simulink model "simulink_4_balloons"  (R2020b)
settings: Solver=VariableStepAuto  StartTime=0.0  StopTime=300  RelTol=1e-3
InitFcn:
  | seed1 = randi(100000);
  | seed2 = randi(200000);
values from neighbouring files (symbols this model uses):
  Cd = 0.418    [sim_4balloon_test.m]
  mb1 = 3/1000    (= 0.003)    [sim_4balloon_test.m]
  mb2 = 3/1000    (= 0.003)    [sim_4balloon_test.m]
  mb3 = 3/1000    (= 0.003)    [sim_4balloon_test.m]
  mb4 = 3/1000    (= 0.003)    [sim_4balloon_test.m]
  nH = x(2)    [sim_4balloon_test.m]
  normalScaling = x(5)    [sim_4balloon_test.m]
  nS = x(3)    [sim_4balloon_test.m]
  nV = x(1)    [sim_4balloon_test.m]
  rb = 80/1000    (= 0.08)    [sim_4balloon_test.m]
  rb1 = 80/1000    (= 0.08)    [sim_4balloon_test.m]
  rb2 = 80/1000    (= 0.08)    [sim_4balloon_test.m]
  rb3 = 80/1000    (= 0.08)    [sim_4balloon_test.m]
  rb4 = 80/1000    (= 0.08)    [sim_4balloon_test.m]
  rn = 125/2000    (= 0.0625)    [sim_4balloon_test.m]
  seedX1 = randi(100000)    [sim_4balloon_test.m]
  seedX2 = randi(100000)    [sim_4balloon_test.m]
  seedX3 = randi(100000)    [sim_4balloon_test.m]
  seedX4 = randi(100000)    [sim_4balloon_test.m]
  seedY1 = randi(100000)    [sim_4balloon_test.m]
  seedY2 = randi(100000)    [sim_4balloon_test.m]
  seedY3 = randi(100000)    [sim_4balloon_test.m]
  seedY4 = randi(100000)    [sim_4balloon_test.m]
  seedZ1 = randi(100000)    [sim_4balloon_test.m]
  seedZ2 = randi(100000)    [sim_4balloon_test.m]
  seedZ3 = randi(100000)    [sim_4balloon_test.m]
  seedZ4 = randi(100000)    [sim_4balloon_test.m]
  theta = x(7)    [sim_4balloon_test.m]
  V0 = x(4)    [sim_4balloon_test.m]
undefined symbols (not defined in the file or in its folder): coefficient_dragq, coefficient_sideforceq
libraries: nesl_utility x41, sm_lib x25, eeGeneralControl x12
(part 2 of 2)

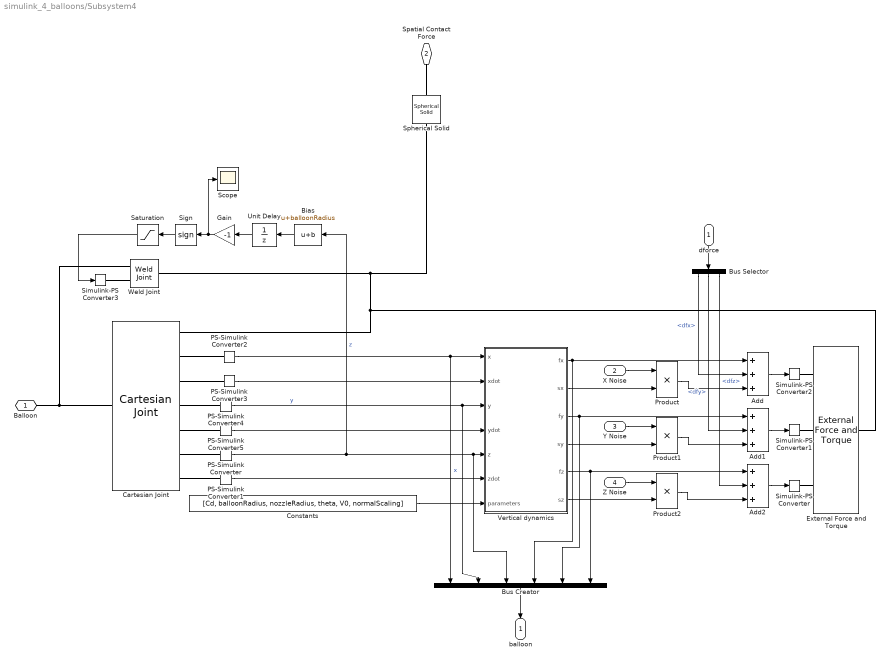
== system simulink_4_balloons/Subsystem4 ==
  dforce : Inport
  X Noise : Inport  Port=2
  Y Noise : Inport  Port=3
  Z Noise : Inport  Port=4
  Add : Sum  Inputs=+++
  Add1 : Sum  Inputs=+++
  Add2 : Sum  Inputs=+++
  Bias : Bias  Bias=balloonRadius
  Bus Creator : BusCreator  Inputs=6
  Bus Selector : BusSelector  OutputSignals=dfx,dfy,dfz
  Cartesian Joint : sm_lib/Joints/Cartesian Joint  JointMode=Normal  SenseConstraintForce=off  SenseConstraintForceX=off  SenseConstraintForceY=off  SenseConstraintForceZ=off  SenseConstraintTorque=off  SenseConstraintTorqueX=off  SenseConstraintTorqueY=off  SenseConstraintTorqueZ=off  SenseTotalForce=off  SenseTotalForceX=off  SenseTotalForceY=off  SenseTotalForceZ=off  SenseTotalTorque=off  SenseTotalTorqueX=off  SenseTotalTorqueY=off  SenseTotalTorqueZ=off  CompositeWrenchDir=FollowerOnBase  CompositeWrenchFrame=BaseFrame  PxEquilibriumPosition=0  PxEquilibriumPositionUnits=m  PxSpringStiffness=0  PxSpringStiffnessUnits=N/m  PxDampingCoefficient=hd  PxDampingCoefficientUnits=N/(m/s)  PxTorqueActuationMode=NoTorque  PxMotionActuationMode=ComputedMotion  PxSensePosition=on  PxSenseVelocity=on  PxSenseAcceleration=off  PxSenseTorqueForce=off  PxSenseLowerLimitTorqueForce=off  PxSenseUpperLimitTorqueForce=off  PxLowerLimitSpecify=off  PxLowerLimitBound=-1  PxLowerLimitBoundUnits=m  PxLowerLimitStiffness=1e6  PxLowerLimitStiffnessUnits=N/m  PxLowerLimitDamping=1e3  PxLowerLimitDampingUnits=N/(m/s)  PxLowerLimitTransitionRegionWidth=1e-4  PxLowerLimitTransitionRegionWidthUnits=m  PxUpperLimitSpecify=off  PxUpperLimitBound=1  PxUpperLimitBoundUnits=m  PxUpperLimitStiffness=1e6  PxUpperLimitStiffnessUnits=N/m  PxUpperLimitDamping=1e3  PxUpperLimitDampingUnits=N/(m/s)  PxUpperLimitTransitionRegionWidth=1e-4  PxUpperLimitTransitionRegionWidthUnits=m  PxPositionTargetSpecify=off  PxPositionTargetPriority=High  PxPositionTargetValue=0  PxPositionTargetValueUnits=m  PxVelocityTargetSpecify=off  PxVelocityTargetPriority=High  PxVelocityTargetValue=0  PxVelocityTargetValueUnits=m/s  PyEquilibriumPosition=0  PyEquilibriumPositionUnits=m  PySpringStiffness=0  PySpringStiffnessUnits=N/m  PyDampingCoefficient=hd  PyDampingCoefficientUnits=N/(m/s)  PyTorqueActuationMode=NoTorque  PyMotionActuationMode=ComputedMotion  PySensePosition=on  PySenseVelocity=on  PySenseAcceleration=off  PySenseTorqueForce=off  PySenseLowerLimitTorqueForce=off  PySenseUpperLimitTorqueForce=off  PyLowerLimitSpecify=off  PyLowerLimitBound=-1  PyLowerLimitBoundUnits=m  PyLowerLimitStiffness=1e6  PyLowerLimitStiffnessUnits=N/m  PyLowerLimitDamping=1e3  PyLowerLimitDampingUnits=N/(m/s)  PyLowerLimitTransitionRegionWidth=1e-4  PyLowerLimitTransitionRegionWidthUnits=m  PyUpperLimitSpecify=off  PyUpperLimitBound=1  PyUpperLimitBoundUnits=m  PyUpperLimitStiffness=1e6  PyUpperLimitStiffnessUnits=N/m  PyUpperLimitDamping=1e3  PyUpperLimitDampingUnits=N/(m/s)  PyUpperLimitTransitionRegionWidth=1e-4  PyUpperLimitTransitionRegionWidthUnits=m  PyPositionTargetSpecify=off  PyPositionTargetPriority=High  PyPositionTargetValue=0  PyPositionTargetValueUnits=m  PyVelocityTargetSpecify=off  PyVelocityTargetPriority=High  PyVelocityTargetValue=0  PyVelocityTargetValueUnits=m/s  PzEquilibriumPosition=0  PzEquilibriumPositionUnits=m  PzSpringStiffness=0  PzSpringStiffnessUnits=N/m  PzDampingCoefficient=hd  PzDampingCoefficientUnits=N/(m/s)  PzTorqueActuationMode=NoTorque  PzMotionActuationMode=ComputedMotion  PzSensePosition=on  PzSenseVelocity=on  PzSenseAcceleration=off  PzSenseTorqueForce=off  PzSenseLowerLimitTorqueForce=off  PzSenseUpperLimitTorqueForce=off  PzLowerLimitSpecify=off  PzLowerLimitBound=0  PzLowerLimitBoundUnits=m  PzLowerLimitStiffness=1e6  PzLowerLimitStiffnessUnits=N/m  PzLowerLimitDamping=1e3  PzLowerLimitDampingUnits=N/(m/s)  PzLowerLimitTransitionRegionWidth=1e-4  PzLowerLimitTransitionRegionWidthUnits=m  PzUpperLimitSpecify=off  PzUpperLimitBound=1  PzUpperLimitBoundUnits=m  PzUpperLimitStiffness=1e6  PzUpperLimitStiffnessUnits=N/m  PzUpperLimitDamping=1e3  PzUpperLimitDampingUnits=N/(m/s)  PzUpperLimitTransitionRegionWidth=1e-4  PzUpperLimitTransitionRegionWidthUnits=m  PzPositionTargetSpecify=on  PzPositionTargetPriority=High  PzPositionTargetValue=initialHeight  PzPositionTargetValueUnits=m  PzVelocityTargetSpecify=on  PzVelocityTargetPriority=High  PzVelocityTargetValue=0  PzVelocityTargetValueUnits=m/s
  Constants : Constant  Value=[Cd, balloonRadius, nozzleRadius, theta, V0, normalScaling]
  External Force and Torque : sm_lib/Forces and Torques/External Force and Torque  ForceResolutionFrame=AttachedFrame  EnableForceX=on  EnableForceY=on  EnableForceZ=on  EnableForce=off  TorqueResolutionFrame=AttachedFrame  EnableTorqueX=off  EnableTorqueY=off  EnableTorqueZ=off  EnableTorque=off
  Gain : Gain  Gain=-1
  PS-Simulink Converter{,1..5} (6 alike) : nesl_utility/PS-Simulink Converter  PhysicalDomain=network_engine_domain  SubClassName=ps_output  LeftPortType=input  RightPortType=output  PseudoPeriodic=off  Frequencies=[]  Unit=inherit  AffineConversion=off
  Product : Product
  Product1 : Product
  Product2 : Product
  Saturation : Saturate  UpperLimit=0  LowerLimit=-1
  Scope : Scope
  Sign : Signum
  Simulink-PS Converter{,1..3} (4 alike) : nesl_utility/Simulink-PS Converter  PhysicalDomain=network_engine_domain  SubClassName=ps_input  LeftPortType=input  RightPortType=output  PseudoPeriodic=off  Frequencies=[]  NoiseDistribution=none  NoiseParameters=[]  Unit=1  AffineConversion=off  FilteringAndDerivatives=provide  SimscapeFilterOrder=1  InputFilterTimeConstant=0.001  UdotUserProvided=0
  Spherical Solid : sm_lib/Body Elements/Spherical Solid  GraphicAmbientColor=[0.15 0.15 0.15 1.0]  BasedOnType=Mass  CenterOfMass=[0 0 0]  CenterOfMassUnits=m  GraphicDiffuseColor=[1.0 1.0 0.0]  Density=1000  DensityUnits=kg/m^3  DoExposeReferenceFrame=on  GraphicEmissiveColor=[0.0 0.0 0.0 1.0]  ExportEntireGeometry=on  SerializedExposedGeometries=<ExposedGeometries><ExposedGeometry><RawGeometryId>entire</RawGeometryId><ExposedGeometryId>G</ExposedGeometryId></ExposedGeometry></ExposedGeometries>  SerializedFrames=<Frames/>  MarkerShape=Sphere  MarkerSize=10  GraphicType=FromGeometry  InertiaType=CalculateFromGeometry  Mass=balloonMass  MassUnits=kg  MomentsOfInertia=[1 1 1]  MomentsOfInertiaUnits=kg*m^2  GraphicOpacity=1.0  ProductsOfInertia=[0 0 0]  ProductsOfInertiaUnits=kg*m^2  GraphicShininess=75  GraphicSpecularColor=[0.5 0.5 0.5 1.0]  SphereRadius=balloonRadius  SphereRadiusUnits=m  GraphicVisPropType=SimpleVisualProperties
  Unit Delay : UnitDelay  InitialCondition=initialHeight+balloonRadius  SampleTime=0.01  HasFrameUpgradeWarning=on
  Vertical dynamics : MATLAB Function  TreatAsAtomicUnit=on
  Weld Joint : sm_lib/Joints/Weld Joint  JointMode=ProvidedByInput  SenseConstraintForce=off  SenseConstraintForceX=off  SenseConstraintForceY=off  SenseConstraintForceZ=off  SenseConstraintTorque=off  SenseConstraintTorqueX=off  SenseConstraintTorqueY=off  SenseConstraintTorqueZ=off  SenseTotalForce=off  SenseTotalForceX=off  SenseTotalForceY=off  SenseTotalForceZ=off  SenseTotalTorque=off  SenseTotalTorqueX=off  SenseTotalTorqueY=off  SenseTotalTorqueZ=off  CompositeWrenchDir=FollowerOnBase  CompositeWrenchFrame=BaseFrame
  Balloon : PMIOPort  Side=Left
  Spatial Contact Force : PMIOPort  Port=2  Side=Left
  balloon : Outport
  wires:
  PS-Simulink Converter4/1 -> Vertical dynamics/3(y), Bus Creator/2  "y"
  PS-Simulink Converter2/1 -> Bus Creator/1, Vertical dynamics/1(x)  "x"
  Gain/1 -> Scope/1, Sign/1
  Unit Delay/1 -> Gain/1
  Sign/1 -> Saturation/1
  Saturation/1 -> Simulink-PS Converter3/1
  Bias/1 -> Unit Delay/1
  Product2/1 -> Add2/3
  Bus Selector/2 -> Add1/2  "<dfy>"
  Bus Selector/3 -> Add2/2  "<dfz>"
  Vertical dynamics/1(fx) -> Add/1, Bus Creator/4
  Vertical dynamics/5(fz) -> Add2/1, Bus Creator/6
  PS-Simulink Converter/1 -> Bus Creator/3, Vertical dynamics/5(z), Bias/1  "z"
  X Noise/1 -> Product/1
  Vertical dynamics/4(sy) -> Product1/2
  Add1/1 -> Simulink-PS Converter1/1
  Add/1 -> Simulink-PS Converter2/1
  Add2/1 -> Simulink-PS Converter/1
  Vertical dynamics/3(fy) -> Add1/1, Bus Creator/5
  Y Noise/1 -> Product1/1
  Vertical dynamics/2(sx) -> Product/2
  Product1/1 -> Add1/3
  Product/1 -> Add/3
  dforce/1 -> Bus Selector/1
  Vertical dynamics/6(sz) -> Product2/2
  Bus Creator/1 -> balloon/1
  Z Noise/1 -> Product2/1
  Bus Selector/1 -> Add/2  "<dfx>"
  PS-Simulink Converter5/1 -> Vertical dynamics/4(ydot)
  PS-Simulink Converter1/1 -> Vertical dynamics/6(zdot)
  PS-Simulink Converter3/1 -> Vertical dynamics/2(xdot)
  Constants/1 -> Vertical dynamics/7(parameters)
  connections:
  PS-Simulink Converter/LConn1 -- Cartesian Joint/RConn6
  PS-Simulink Converter2/LConn1 -- Cartesian Joint/RConn2
  Weld Joint/RConn1 -- Spherical Solid/RConn1 -- External Force and Torque/RConn1 -- Cartesian Joint/RConn1
  Cartesian Joint/LConn1 -- Weld Joint/LConn1 -- Balloon/RConn1
  PS-Simulink Converter5/LConn1 -- Cartesian Joint/RConn5
  Cartesian Joint/RConn4 -- PS-Simulink Converter4/LConn1
  PS-Simulink Converter3/LConn1 -- Cartesian Joint/RConn3
  PS-Simulink Converter1/LConn1 -- Cartesian Joint/RConn7
  Simulink-PS Converter3/RConn1 -- Weld Joint/LConn2
  Spatial Contact Force/RConn1 -- Spherical Solid/LConn1
  Simulink-PS Converter1/RConn1 -- External Force and Torque/LConn2
  Simulink-PS Converter/RConn1 -- External Force and Torque/LConn3
  External Force and Torque/LConn1 -- Simulink-PS Converter2/RConn1

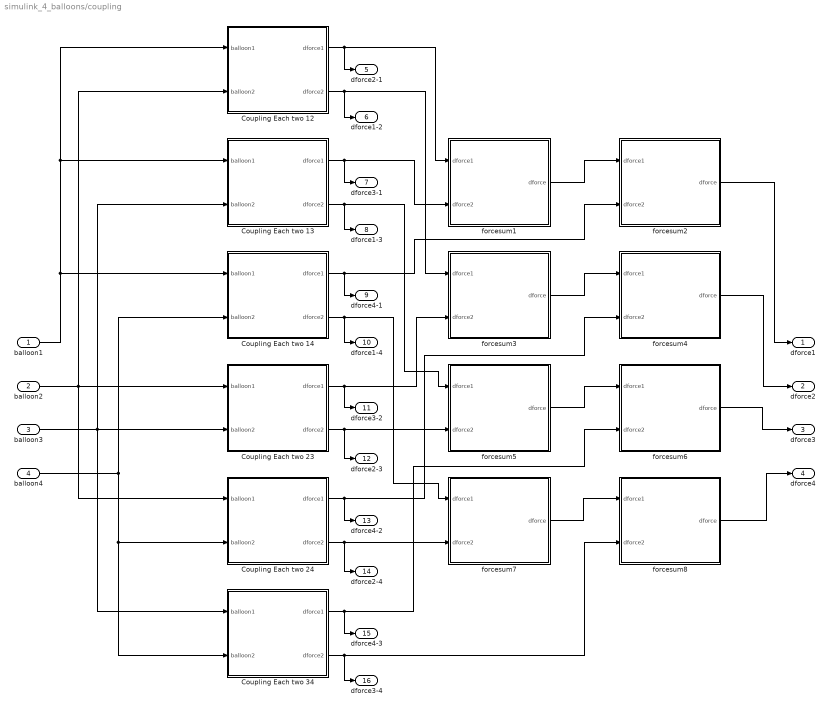
== system simulink_4_balloons/coupling ==
  balloon1 : Inport
  balloon2 : Inport  Port=2
  balloon3 : Inport  Port=3
  balloon4 : Inport  Port=4
  Coupling Each two 12 : Subsystem
  Coupling Each two 13 : Subsystem
  Coupling Each two 14 : Subsystem
  Coupling Each two 23 : Subsystem
  Coupling Each two 24 : Subsystem
  Coupling Each two 34 : Subsystem
  forcesum1 : Subsystem
  forcesum2 : Subsystem
  forcesum3 : Subsystem
  forcesum4 : Subsystem
  forcesum5 : Subsystem
  forcesum6 : Subsystem
  forcesum7 : Subsystem
  forcesum8 : Subsystem
  dforce1 : Outport
  dforce2 : Outport  Port=2
  dforce3 : Outport  Port=3
  dforce4 : Outport  Port=4
  dforce2-1 : Outport  Port=5
  dforce1-2 : Outport  Port=6
  dforce3-1 : Outport  Port=7
  dforce1-3 : Outport  Port=8
  dforce4-1 : Outport  Port=9
  dforce1-4 : Outport  Port=10
  dforce3-2 : Outport  Port=11
  dforce2-3 : Outport  Port=12
  dforce4-2 : Outport  Port=13
  dforce2-4 : Outport  Port=14
  dforce4-3 : Outport  Port=15
  dforce3-4 : Outport  Port=16
  wires:
  balloon1/1 -> Coupling Each two 14/1(balloon1), Coupling Each two 12/1(balloon1), Coupling Each two 13/1(balloon1)
  balloon2/1 -> Coupling Each two 24/1(balloon1), Coupling Each two 12/2(balloon2), Coupling Each two 23/1(balloon1)
  balloon3/1 -> Coupling Each two 23/2(balloon2), Coupling Each two 34/1(balloon1), Coupling Each two 13/2(balloon2)
  balloon4/1 -> Coupling Each two 24/2(balloon2), Coupling Each two 34/2(balloon2), Coupling Each two 14/2(balloon2)
  Coupling Each two 12/1(dforce1) -> dforce2-1/1, forcesum1/1(dforce1)
  Coupling Each two 13/1(dforce1) -> dforce3-1/1, forcesum1/2(dforce2)
  forcesum1/1(dforce) -> forcesum2/1(dforce1)
  Coupling Each two 14/1(dforce1) -> dforce4-1/1, forcesum2/2(dforce2)
  forcesum2/1(dforce) -> dforce1/1
  Coupling Each two 12/2(dforce2) -> dforce1-2/1, forcesum3/1(dforce1)
  Coupling Each two 23/1(dforce1) -> dforce3-2/1, forcesum3/2(dforce2)
  Coupling Each two 24/1(dforce1) -> dforce4-2/1, forcesum4/2(dforce2)
  forcesum3/1(dforce) -> forcesum4/1(dforce1)
  forcesum4/1(dforce) -> dforce2/1
  Coupling Each two 13/2(dforce2) -> dforce1-3/1, forcesum5/1(dforce1)
  Coupling Each two 23/2(dforce2) -> dforce2-3/1, forcesum5/2(dforce2)
  Coupling Each two 34/1(dforce1) -> dforce4-3/1, forcesum6/2(dforce2)
  forcesum5/1(dforce) -> forcesum6/1(dforce1)
  forcesum6/1(dforce) -> dforce3/1
  Coupling Each two 34/2(dforce2) -> dforce3-4/1, forcesum8/2(dforce2)
  Coupling Each two 24/2(dforce2) -> dforce2-4/1, forcesum7/2(dforce2)
  Coupling Each two 14/2(dforce2) -> dforce1-4/1, forcesum7/1(dforce1)
  forcesum7/1(dforce) -> forcesum8/1(dforce1)
  forcesum8/1(dforce) -> dforce4/1

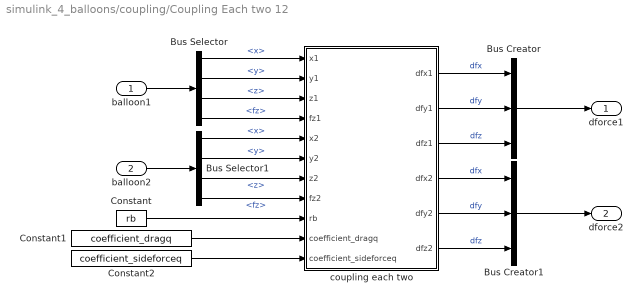
== system simulink_4_balloons/coupling/Coupling Each two 12 ==
  balloon1 : Inport
  balloon2 : Inport  Port=2
  Bus Creator : BusCreator  Inputs=3
  Bus Creator1 : BusCreator  Inputs=3
  Bus Selector : BusSelector  OutputSignals=x,y,z,fz
  Bus Selector1 : BusSelector  OutputSignals=x,y,z,fz
  Constant : Constant  Value=rb
  Constant1 : Constant  Value=coefficient_dragq
  Constant2 : Constant  Value=coefficient_sideforceq
  coupling each two : MATLAB Function  TreatAsAtomicUnit=on
  dforce1 : Outport
  dforce2 : Outport  Port=2
  wires:
  coupling each two/3(dfz1) -> Bus Creator/3  "dfz"
  coupling each two/2(dfy1) -> Bus Creator/2  "dfy"
  coupling each two/1(dfx1) -> Bus Creator/1  "dfx"
  Bus Creator/1 -> dforce1/1
  coupling each two/4(dfx2) -> Bus Creator1/1  "dfx"
  coupling each two/5(dfy2) -> Bus Creator1/2  "dfy"
  coupling each two/6(dfz2) -> Bus Creator1/3  "dfz"
  Bus Creator1/1 -> dforce2/1
  balloon1/1 -> Bus Selector/1
  Bus Selector/4 -> coupling each two/4(fz1)  "<fz>"
  Bus Selector/1 -> coupling each two/1(x1)  "<x>"
  Bus Selector/2 -> coupling each two/2(y1)  "<y>"
  Bus Selector/3 -> coupling each two/3(z1)  "<z>"
  balloon2/1 -> Bus Selector1/1
  Bus Selector1/1 -> coupling each two/5(x2)  "<x>"
  Bus Selector1/2 -> coupling each two/6(y2)  "<y>"
  Bus Selector1/3 -> coupling each two/7(z2)  "<z>"
  Bus Selector1/4 -> coupling each two/8(fz2)  "<fz>"
  Constant/1 -> coupling each two/9(rb)
  Constant1/1 -> coupling each two/10(coefficient_dragq)
  Constant2/1 -> coupling each two/11(coefficient_sideforceq)

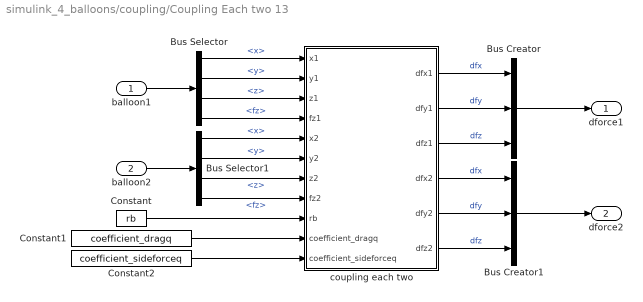
== system simulink_4_balloons/coupling/Coupling Each two 13 ==
  balloon1 : Inport
  balloon2 : Inport  Port=2
  Bus Creator : BusCreator  Inputs=3
  Bus Creator1 : BusCreator  Inputs=3
  Bus Selector : BusSelector  OutputSignals=x,y,z,fz
  Bus Selector1 : BusSelector  OutputSignals=x,y,z,fz
  Constant : Constant  Value=rb
  Constant1 : Constant  Value=coefficient_dragq
  Constant2 : Constant  Value=coefficient_sideforceq
  coupling each two : MATLAB Function  TreatAsAtomicUnit=on
  dforce1 : Outport
  dforce2 : Outport  Port=2
  wires:
  coupling each two/3(dfz1) -> Bus Creator/3  "dfz"
  coupling each two/2(dfy1) -> Bus Creator/2  "dfy"
  coupling each two/1(dfx1) -> Bus Creator/1  "dfx"
  Bus Creator/1 -> dforce1/1
  coupling each two/4(dfx2) -> Bus Creator1/1  "dfx"
  coupling each two/5(dfy2) -> Bus Creator1/2  "dfy"
  coupling each two/6(dfz2) -> Bus Creator1/3  "dfz"
  Bus Creator1/1 -> dforce2/1
  balloon1/1 -> Bus Selector/1
  Bus Selector/4 -> coupling each two/4(fz1)  "<fz>"
  Bus Selector/1 -> coupling each two/1(x1)  "<x>"
  Bus Selector/2 -> coupling each two/2(y1)  "<y>"
  Bus Selector/3 -> coupling each two/3(z1)  "<z>"
  balloon2/1 -> Bus Selector1/1
  Bus Selector1/1 -> coupling each two/5(x2)  "<x>"
  Bus Selector1/2 -> coupling each two/6(y2)  "<y>"
  Bus Selector1/3 -> coupling each two/7(z2)  "<z>"
  Bus Selector1/4 -> coupling each two/8(fz2)  "<fz>"
  Constant/1 -> coupling each two/9(rb)
  Constant1/1 -> coupling each two/10(coefficient_dragq)
  Constant2/1 -> coupling each two/11(coefficient_sideforceq)

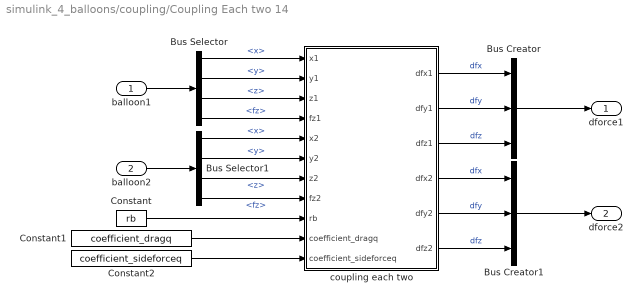
== system simulink_4_balloons/coupling/Coupling Each two 14 ==
  balloon1 : Inport
  balloon2 : Inport  Port=2
  Bus Creator : BusCreator  Inputs=3
  Bus Creator1 : BusCreator  Inputs=3
  Bus Selector : BusSelector  OutputSignals=x,y,z,fz
  Bus Selector1 : BusSelector  OutputSignals=x,y,z,fz
  Constant : Constant  Value=rb
  Constant1 : Constant  Value=coefficient_dragq
  Constant2 : Constant  Value=coefficient_sideforceq
  coupling each two : MATLAB Function  TreatAsAtomicUnit=on
  dforce1 : Outport
  dforce2 : Outport  Port=2
  wires:
  coupling each two/3(dfz1) -> Bus Creator/3  "dfz"
  coupling each two/2(dfy1) -> Bus Creator/2  "dfy"
  coupling each two/1(dfx1) -> Bus Creator/1  "dfx"
  Bus Creator/1 -> dforce1/1
  coupling each two/4(dfx2) -> Bus Creator1/1  "dfx"
  coupling each two/5(dfy2) -> Bus Creator1/2  "dfy"
  coupling each two/6(dfz2) -> Bus Creator1/3  "dfz"
  Bus Creator1/1 -> dforce2/1
  balloon1/1 -> Bus Selector/1
  Bus Selector/4 -> coupling each two/4(fz1)  "<fz>"
  Bus Selector/1 -> coupling each two/1(x1)  "<x>"
  Bus Selector/2 -> coupling each two/2(y1)  "<y>"
  Bus Selector/3 -> coupling each two/3(z1)  "<z>"
  balloon2/1 -> Bus Selector1/1
  Bus Selector1/1 -> coupling each two/5(x2)  "<x>"
  Bus Selector1/2 -> coupling each two/6(y2)  "<y>"
  Bus Selector1/3 -> coupling each two/7(z2)  "<z>"
  Bus Selector1/4 -> coupling each two/8(fz2)  "<fz>"
  Constant/1 -> coupling each two/9(rb)
  Constant1/1 -> coupling each two/10(coefficient_dragq)
  Constant2/1 -> coupling each two/11(coefficient_sideforceq)

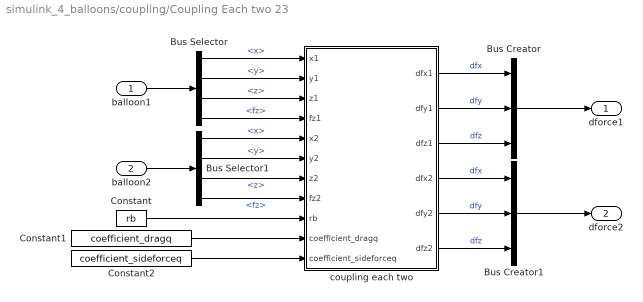
== system simulink_4_balloons/coupling/Coupling Each two 23 ==
  balloon1 : Inport
  balloon2 : Inport  Port=2
  Bus Creator : BusCreator  Inputs=3
  Bus Creator1 : BusCreator  Inputs=3
  Bus Selector : BusSelector  OutputSignals=x,y,z,fz
  Bus Selector1 : BusSelector  OutputSignals=x,y,z,fz
  Constant : Constant  Value=rb
  Constant1 : Constant  Value=coefficient_dragq
  Constant2 : Constant  Value=coefficient_sideforceq
  coupling each two : MATLAB Function  TreatAsAtomicUnit=on
  dforce1 : Outport
  dforce2 : Outport  Port=2
  wires:
  coupling each two/3(dfz1) -> Bus Creator/3  "dfz"
  coupling each two/2(dfy1) -> Bus Creator/2  "dfy"
  coupling each two/1(dfx1) -> Bus Creator/1  "dfx"
  Bus Creator/1 -> dforce1/1
  coupling each two/4(dfx2) -> Bus Creator1/1  "dfx"
  coupling each two/5(dfy2) -> Bus Creator1/2  "dfy"
  coupling each two/6(dfz2) -> Bus Creator1/3  "dfz"
  Bus Creator1/1 -> dforce2/1
  balloon1/1 -> Bus Selector/1
  Bus Selector/4 -> coupling each two/4(fz1)  "<fz>"
  Bus Selector/1 -> coupling each two/1(x1)  "<x>"
  Bus Selector/2 -> coupling each two/2(y1)  "<y>"
  Bus Selector/3 -> coupling each two/3(z1)  "<z>"
  balloon2/1 -> Bus Selector1/1
  Bus Selector1/1 -> coupling each two/5(x2)  "<x>"
  Bus Selector1/2 -> coupling each two/6(y2)  "<y>"
  Bus Selector1/3 -> coupling each two/7(z2)  "<z>"
  Bus Selector1/4 -> coupling each two/8(fz2)  "<fz>"
  Constant/1 -> coupling each two/9(rb)
  Constant1/1 -> coupling each two/10(coefficient_dragq)
  Constant2/1 -> coupling each two/11(coefficient_sideforceq)

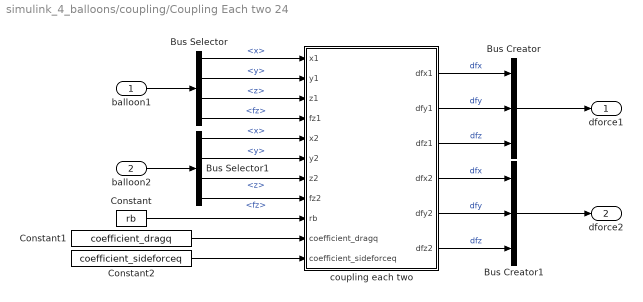
== system simulink_4_balloons/coupling/Coupling Each two 24 ==
  balloon1 : Inport
  balloon2 : Inport  Port=2
  Bus Creator : BusCreator  Inputs=3
  Bus Creator1 : BusCreator  Inputs=3
  Bus Selector : BusSelector  OutputSignals=x,y,z,fz
  Bus Selector1 : BusSelector  OutputSignals=x,y,z,fz
  Constant : Constant  Value=rb
  Constant1 : Constant  Value=coefficient_dragq
  Constant2 : Constant  Value=coefficient_sideforceq
  coupling each two : MATLAB Function  TreatAsAtomicUnit=on
  dforce1 : Outport
  dforce2 : Outport  Port=2
  wires:
  coupling each two/3(dfz1) -> Bus Creator/3  "dfz"
  coupling each two/2(dfy1) -> Bus Creator/2  "dfy"
  coupling each two/1(dfx1) -> Bus Creator/1  "dfx"
  Bus Creator/1 -> dforce1/1
  coupling each two/4(dfx2) -> Bus Creator1/1  "dfx"
  coupling each two/5(dfy2) -> Bus Creator1/2  "dfy"
  coupling each two/6(dfz2) -> Bus Creator1/3  "dfz"
  Bus Creator1/1 -> dforce2/1
  balloon1/1 -> Bus Selector/1
  Bus Selector/4 -> coupling each two/4(fz1)  "<fz>"
  Bus Selector/1 -> coupling each two/1(x1)  "<x>"
  Bus Selector/2 -> coupling each two/2(y1)  "<y>"
  Bus Selector/3 -> coupling each two/3(z1)  "<z>"
  balloon2/1 -> Bus Selector1/1
  Bus Selector1/1 -> coupling each two/5(x2)  "<x>"
  Bus Selector1/2 -> coupling each two/6(y2)  "<y>"
  Bus Selector1/3 -> coupling each two/7(z2)  "<z>"
  Bus Selector1/4 -> coupling each two/8(fz2)  "<fz>"
  Constant/1 -> coupling each two/9(rb)
  Constant1/1 -> coupling each two/10(coefficient_dragq)
  Constant2/1 -> coupling each two/11(coefficient_sideforceq)

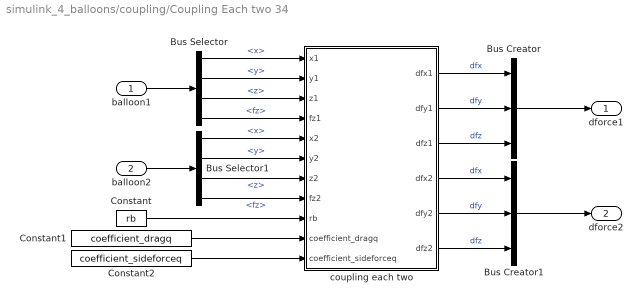
== system simulink_4_balloons/coupling/Coupling Each two 34 ==
  balloon1 : Inport
  balloon2 : Inport  Port=2
  Bus Creator : BusCreator  Inputs=3
  Bus Creator1 : BusCreator  Inputs=3
  Bus Selector : BusSelector  OutputSignals=x,y,z,fz
  Bus Selector1 : BusSelector  OutputSignals=x,y,z,fz
  Constant : Constant  Value=rb
  Constant1 : Constant  Value=coefficient_dragq
  Constant2 : Constant  Value=coefficient_sideforceq
  coupling each two : MATLAB Function  TreatAsAtomicUnit=on
  dforce1 : Outport
  dforce2 : Outport  Port=2
  wires:
  coupling each two/3(dfz1) -> Bus Creator/3  "dfz"
  coupling each two/2(dfy1) -> Bus Creator/2  "dfy"
  coupling each two/1(dfx1) -> Bus Creator/1  "dfx"
  Bus Creator/1 -> dforce1/1
  coupling each two/4(dfx2) -> Bus Creator1/1  "dfx"
  coupling each two/5(dfy2) -> Bus Creator1/2  "dfy"
  coupling each two/6(dfz2) -> Bus Creator1/3  "dfz"
  Bus Creator1/1 -> dforce2/1
  balloon1/1 -> Bus Selector/1
  Bus Selector/4 -> coupling each two/4(fz1)  "<fz>"
  Bus Selector/1 -> coupling each two/1(x1)  "<x>"
  Bus Selector/2 -> coupling each two/2(y1)  "<y>"
  Bus Selector/3 -> coupling each two/3(z1)  "<z>"
  balloon2/1 -> Bus Selector1/1
  Bus Selector1/1 -> coupling each two/5(x2)  "<x>"
  Bus Selector1/2 -> coupling each two/6(y2)  "<y>"
  Bus Selector1/3 -> coupling each two/7(z2)  "<z>"
  Bus Selector1/4 -> coupling each two/8(fz2)  "<fz>"
  Constant/1 -> coupling each two/9(rb)
  Constant1/1 -> coupling each two/10(coefficient_dragq)
  Constant2/1 -> coupling each two/11(coefficient_sideforceq)

== system simulink_4_balloons/coupling/forcesum1 ==
  dforce1 : Inport
  dforce2 : Inport  Port=2
  Bus Creator : BusCreator  Inputs=3
  Bus Selector : BusSelector  OutputSignals=dfx,dfy,dfz
  Bus Selector1 : BusSelector  OutputSignals=dfx,dfy,dfz
  Sum : Sum
  Sum1 : Sum
  Sum2 : Sum
  dforce : Outport
  wires:
  dforce1/1 -> Bus Selector/1
  dforce2/1 -> Bus Selector1/1
  Bus Creator/1 -> dforce/1
  Bus Selector/1 -> Sum/1  "<dfx>"
  Bus Selector1/1 -> Sum/2  "<dfx>"
  Sum/1 -> Bus Creator/1  "dfx"
  Bus Selector/2 -> Sum1/1  "<dfy>"
  Bus Selector/3 -> Sum2/1  "<dfz>"
  Bus Selector1/2 -> Sum1/2  "<dfy>"
  Bus Selector1/3 -> Sum2/2  "<dfz>"
  Sum1/1 -> Bus Creator/2  "dfy"
  Sum2/1 -> Bus Creator/3  "dfz"

== system simulink_4_balloons/coupling/forcesum2 ==
  dforce1 : Inport
  dforce2 : Inport  Port=2
  Bus Creator : BusCreator  Inputs=3
  Bus Selector : BusSelector  OutputSignals=dfx,dfy,dfz
  Bus Selector1 : BusSelector  OutputSignals=dfx,dfy,dfz
  Sum : Sum
  Sum1 : Sum
  Sum2 : Sum
  dforce : Outport
  wires:
  dforce1/1 -> Bus Selector/1
  dforce2/1 -> Bus Selector1/1
  Bus Creator/1 -> dforce/1
  Bus Selector/1 -> Sum/1  "<dfx>"
  Bus Selector1/1 -> Sum/2  "<dfx>"
  Sum/1 -> Bus Creator/1  "dfx"
  Bus Selector/2 -> Sum1/1  "<dfy>"
  Bus Selector/3 -> Sum2/1  "<dfz>"
  Bus Selector1/2 -> Sum1/2  "<dfy>"
  Bus Selector1/3 -> Sum2/2  "<dfz>"
  Sum1/1 -> Bus Creator/2  "dfy"
  Sum2/1 -> Bus Creator/3  "dfz"

== system simulink_4_balloons/coupling/forcesum3 ==
  dforce1 : Inport
  dforce2 : Inport  Port=2
  Bus Creator : BusCreator  Inputs=3
  Bus Selector : BusSelector  OutputSignals=dfx,dfy,dfz
  Bus Selector1 : BusSelector  OutputSignals=dfx,dfy,dfz
  Sum : Sum
  Sum1 : Sum
  Sum2 : Sum
  dforce : Outport
  wires:
  dforce1/1 -> Bus Selector/1
  dforce2/1 -> Bus Selector1/1
  Bus Creator/1 -> dforce/1
  Bus Selector/1 -> Sum/1  "<dfx>"
  Bus Selector1/1 -> Sum/2  "<dfx>"
  Sum/1 -> Bus Creator/1  "dfx"
  Bus Selector/2 -> Sum1/1  "<dfy>"
  Bus Selector/3 -> Sum2/1  "<dfz>"
  Bus Selector1/2 -> Sum1/2  "<dfy>"
  Bus Selector1/3 -> Sum2/2  "<dfz>"
  Sum1/1 -> Bus Creator/2  "dfy"
  Sum2/1 -> Bus Creator/3  "dfz"

== system simulink_4_balloons/coupling/forcesum4 ==
  dforce1 : Inport
  dforce2 : Inport  Port=2
  Bus Creator : BusCreator  Inputs=3
  Bus Selector : BusSelector  OutputSignals=dfx,dfy,dfz
  Bus Selector1 : BusSelector  OutputSignals=dfx,dfy,dfz
  Sum : Sum
  Sum1 : Sum
  Sum2 : Sum
  dforce : Outport
  wires:
  dforce1/1 -> Bus Selector/1
  dforce2/1 -> Bus Selector1/1
  Bus Creator/1 -> dforce/1
  Bus Selector/1 -> Sum/1  "<dfx>"
  Bus Selector1/1 -> Sum/2  "<dfx>"
  Sum/1 -> Bus Creator/1  "dfx"
  Bus Selector/2 -> Sum1/1  "<dfy>"
  Bus Selector/3 -> Sum2/1  "<dfz>"
  Bus Selector1/2 -> Sum1/2  "<dfy>"
  Bus Selector1/3 -> Sum2/2  "<dfz>"
  Sum1/1 -> Bus Creator/2  "dfy"
  Sum2/1 -> Bus Creator/3  "dfz"

== system simulink_4_balloons/coupling/forcesum5 ==
  dforce1 : Inport
  dforce2 : Inport  Port=2
  Bus Creator : BusCreator  Inputs=3
  Bus Selector : BusSelector  OutputSignals=dfx,dfy,dfz
  Bus Selector1 : BusSelector  OutputSignals=dfx,dfy,dfz
  Sum : Sum
  Sum1 : Sum
  Sum2 : Sum
  dforce : Outport
  wires:
  dforce1/1 -> Bus Selector/1
  dforce2/1 -> Bus Selector1/1
  Bus Creator/1 -> dforce/1
  Bus Selector/1 -> Sum/1  "<dfx>"
  Bus Selector1/1 -> Sum/2  "<dfx>"
  Sum/1 -> Bus Creator/1  "dfx"
  Bus Selector/2 -> Sum1/1  "<dfy>"
  Bus Selector/3 -> Sum2/1  "<dfz>"
  Bus Selector1/2 -> Sum1/2  "<dfy>"
  Bus Selector1/3 -> Sum2/2  "<dfz>"
  Sum1/1 -> Bus Creator/2  "dfy"
  Sum2/1 -> Bus Creator/3  "dfz"

== system simulink_4_balloons/coupling/forcesum6 ==
  dforce1 : Inport
  dforce2 : Inport  Port=2
  Bus Creator : BusCreator  Inputs=3
  Bus Selector : BusSelector  OutputSignals=dfx,dfy,dfz
  Bus Selector1 : BusSelector  OutputSignals=dfx,dfy,dfz
  Sum : Sum
  Sum1 : Sum
  Sum2 : Sum
  dforce : Outport
  wires:
  dforce1/1 -> Bus Selector/1
  dforce2/1 -> Bus Selector1/1
  Bus Creator/1 -> dforce/1
  Bus Selector/1 -> Sum/1  "<dfx>"
  Bus Selector1/1 -> Sum/2  "<dfx>"
  Sum/1 -> Bus Creator/1  "dfx"
  Bus Selector/2 -> Sum1/1  "<dfy>"
  Bus Selector/3 -> Sum2/1  "<dfz>"
  Bus Selector1/2 -> Sum1/2  "<dfy>"
  Bus Selector1/3 -> Sum2/2  "<dfz>"
  Sum1/1 -> Bus Creator/2  "dfy"
  Sum2/1 -> Bus Creator/3  "dfz"

== system simulink_4_balloons/coupling/forcesum7 ==
  dforce1 : Inport
  dforce2 : Inport  Port=2
  Bus Creator : BusCreator  Inputs=3
  Bus Selector : BusSelector  OutputSignals=dfx,dfy,dfz
  Bus Selector1 : BusSelector  OutputSignals=dfx,dfy,dfz
  Sum : Sum
  Sum1 : Sum
  Sum2 : Sum
  dforce : Outport
  wires:
  dforce1/1 -> Bus Selector/1
  dforce2/1 -> Bus Selector1/1
  Bus Creator/1 -> dforce/1
  Bus Selector/1 -> Sum/1  "<dfx>"
  Bus Selector1/1 -> Sum/2  "<dfx>"
  Sum/1 -> Bus Creator/1  "dfx"
  Bus Selector/2 -> Sum1/1  "<dfy>"
  Bus Selector/3 -> Sum2/1  "<dfz>"
  Bus Selector1/2 -> Sum1/2  "<dfy>"
  Bus Selector1/3 -> Sum2/2  "<dfz>"
  Sum1/1 -> Bus Creator/2  "dfy"
  Sum2/1 -> Bus Creator/3  "dfz"

== system simulink_4_balloons/coupling/forcesum8 ==
  dforce1 : Inport
  dforce2 : Inport  Port=2
  Bus Creator : BusCreator  Inputs=3
  Bus Selector : BusSelector  OutputSignals=dfx,dfy,dfz
  Bus Selector1 : BusSelector  OutputSignals=dfx,dfy,dfz
  Sum : Sum
  Sum1 : Sum
  Sum2 : Sum
  dforce : Outport
  wires:
  dforce1/1 -> Bus Selector/1
  dforce2/1 -> Bus Selector1/1
  Bus Creator/1 -> dforce/1
  Bus Selector/1 -> Sum/1  "<dfx>"
  Bus Selector1/1 -> Sum/2  "<dfx>"
  Sum/1 -> Bus Creator/1  "dfx"
  Bus Selector/2 -> Sum1/1  "<dfy>"
  Bus Selector/3 -> Sum2/1  "<dfz>"
  Bus Selector1/2 -> Sum1/2  "<dfy>"
  Bus Selector1/3 -> Sum2/2  "<dfz>"
  Sum1/1 -> Bus Creator/2  "dfy"
  Sum2/1 -> Bus Creator/3  "dfz"

== matlab function simulink_4_balloons/Subsystem4/Vertical dynamics ==
  data: fx output; sx output; fy output; sy output; x input; xdot input; y input; ydot input; z input; fz output; zdot input; parameters input; sz output
function [fx,sx,fy,sy,fz,sz] = fcn(x,xdot,y,ydot,z,zdot,parameters)

Cd = parameters(1);
rb = parameters(2);
rn = parameters(3);
theta = deg2rad(parameters(4)); 
V0 = parameters(5); 
normalScaling = parameters(6); 

%% Vertical forces

%flow radius
rFlow = rn+z*tan(theta);

%Peak flow velocity
meanFlowVelocity = V0*rn^2/(rFlow)^2;

%Velocity under ball
vFlowActual = flowSpeed(meanFlowVelocity,normalScaling*rFlow,x,y);

%Relative
relativeVelocity = vFlowActual - zdot;

%Force
fz = sign(relativeVelocity)*0.5*Cd*pi*rb^2*1.22*relativeVelocity^2;



%% Horizontal XY forces
% Bernoulli's Principle
if x == 0 && y == 0
    fx = 0;
    fy = 0;
else
    direction = [x y];
    distance = norm(direction);
    one_direction = direction/distance;
    inner_position = (distance - rb)*one_direction;
    outer_position = (distance + rb)*one_direction;
    vInner = flowSpeed(meanFlowVelocity,normalScaling*rFlow,inner_position(1),inner_position(2));
    vOuter = flowSpeed(meanFlowVelocity,normalScaling*rFlow,outer_position(1),outer_position(2));
    fH = 0.5*1.22*(vOuter^2 - vInner^2)*pi*rb^2*one_direction;
    fx = fH(1);
    fy = fH(2);
end
% Drag
if xdot == 0 && ydot == 0
else
    vxy = [xdot ydot];
    dragH = 0.5*Cd*pi*rb^2*1.22*(xdot^2 + ydot^2)*vxy/norm(vxy);
    fx = fx - dragH(1);
    fy = fy - dragH(2);
end

%% Force scalings
sx = flowSpeed(meanFlowVelocity,normalScaling*rFlow,x,0)/flowSpeed(meanFlowVelocity,rFlow,0,0);
sy = flowSpeed(meanFlowVelocity,normalScaling*rFlow,0,y)/flowSpeed(meanFlowVelocity,rFlow,0,0);
sz = flowSpeed(meanFlowVelocity,normalScaling*rFlow,x,y)/flowSpeed(meanFlowVelocity,rFlow,0,0);

== matlab function simulink_4_balloons/coupling/Coupling Each two 13/coupling each two ==
  data: x1 input; dfx1 output; y1 input; dfy1 output; dfz1 output; dfx2 output; dfy2 output; dfz2 output; z1 input; fz1 input; x2 input; y2 input; z2 input; fz2 input; rb input; coefficient_dragq input; coefficient_sideforceq input
function [dfx1,dfy1,dfz1,dfx2,dfy2,dfz2] = fcn(x1, y1, z1, fz1, x2, y2, z2, fz2, rb, coefficient_dragq, coefficient_sideforceq)
    % set vector between balloons and z axis
    vector = [x2-x1 y2-y1 z2-z1];
    vectorz = [0 0 1];
    % distance of balloons
    R = norm(vector)/rb/2;
    
    if R >5 || R < 1 % too far
        dfx1 = 0;
        dfy1 = 0;
        dfz1 = 0;
        dfx2 = 0;
        dfy2 = 0;
        dfz2 = 0;
    else % fit curves
        theta2 = acos(dot(vector,vectorz)/(norm(vector)*norm(vectorz)))/pi*180;
        theta1 = 180 - theta2;
        hvector2 = [x2-x1 y2-y1];
        hvector1 = [x1-x2 y1-y2];
        thetaq1 = floor((theta1-0)/1) + 1;
        thetaq2 = floor((theta2-0)/1) + 1;
        Rq1 = floor((R-1)/0.01) + 1;
        Rq2 = floor((R-1)/0.01) + 1;

        % drag fit
        dfz1 = (coefficient_dragq(thetaq1, Rq1) - 1)*fz1;
        dfz2 = (coefficient_dragq(thetaq2, Rq2) - 1)*fz2;

        % sideforce fit
        if norm(hvector1) == 0 % no sideforce
            dfx1 = 0;
            dfy1 = 0;
            dfx2 = 0;
            dfy2 = 0;
        else
            dsideforce1 = coefficient_sideforceq(thetaq1, Rq1)*fz1*hvector1/norm(hvector1);
            dsideforce2 = coefficient_sideforceq(thetaq2, Rq2)*fz2*hvector2/norm(hvector2);
            dfx1 = dsideforce1(1);
            dfy1 = dsideforce1(2);
            dfx2 = dsideforce2(1);
            dfy2 = dsideforce2(2);
        end
    end
end

== matlab function simulink_4_balloons/coupling/Coupling Each two 14/coupling each two ==
  data: x1 input; dfx1 output; y1 input; dfy1 output; dfz1 output; dfx2 output; dfy2 output; dfz2 output; z1 input; fz1 input; x2 input; y2 input; z2 input; fz2 input; rb input; coefficient_dragq input; coefficient_sideforceq input
function [dfx1,dfy1,dfz1,dfx2,dfy2,dfz2] = fcn(x1, y1, z1, fz1, x2, y2, z2, fz2, rb, coefficient_dragq, coefficient_sideforceq)
    % set vector between balloons and z axis
    vector = [x2-x1 y2-y1 z2-z1];
    vectorz = [0 0 1];
    % distance of balloons
    R = norm(vector)/rb/2;
    
    if R >5 || R < 1 % too far
        dfx1 = 0;
        dfy1 = 0;
        dfz1 = 0;
        dfx2 = 0;
        dfy2 = 0;
        dfz2 = 0;
    else % fit curves
        theta2 = acos(dot(vector,vectorz)/(norm(vector)*norm(vectorz)))/pi*180;
        theta1 = 180 - theta2;
        hvector2 = [x2-x1 y2-y1];
        hvector1 = [x1-x2 y1-y2];
        thetaq1 = floor((theta1-0)/1) + 1;
        thetaq2 = floor((theta2-0)/1) + 1;
        Rq1 = floor((R-1)/0.01) + 1;
        Rq2 = floor((R-1)/0.01) + 1;

        % drag fit
        dfz1 = (coefficient_dragq(thetaq1, Rq1) - 1)*fz1;
        dfz2 = (coefficient_dragq(thetaq2, Rq2) - 1)*fz2;

        % sideforce fit
        if norm(hvector1) == 0 % no sideforce
            dfx1 = 0;
            dfy1 = 0;
            dfx2 = 0;
            dfy2 = 0;
        else
            dsideforce1 = coefficient_sideforceq(thetaq1, Rq1)*fz1*hvector1/norm(hvector1);
            dsideforce2 = coefficient_sideforceq(thetaq2, Rq2)*fz2*hvector2/norm(hvector2);
            dfx1 = dsideforce1(1);
            dfy1 = dsideforce1(2);
            dfx2 = dsideforce2(1);
            dfy2 = dsideforce2(2);
        end
    end
end

== matlab function simulink_4_balloons/coupling/Coupling Each two 23/coupling each two ==
  data: x1 input; dfx1 output; y1 input; dfy1 output; dfz1 output; dfx2 output; dfy2 output; dfz2 output; z1 input; fz1 input; x2 input; y2 input; z2 input; fz2 input; rb input; coefficient_dragq input; coefficient_sideforceq input
function [dfx1,dfy1,dfz1,dfx2,dfy2,dfz2] = fcn(x1, y1, z1, fz1, x2, y2, z2, fz2, rb, coefficient_dragq, coefficient_sideforceq)
    % set vector between balloons and z axis
    vector = [x2-x1 y2-y1 z2-z1];
    vectorz = [0 0 1];
    % distance of balloons
    R = norm(vector)/rb/2;
    
    if R >5 || R < 1 % too far
        dfx1 = 0;
        dfy1 = 0;
        dfz1 = 0;
        dfx2 = 0;
        dfy2 = 0;
        dfz2 = 0;
    else % fit curves
        theta2 = acos(dot(vector,vectorz)/(norm(vector)*norm(vectorz)))/pi*180;
        theta1 = 180 - theta2;
        hvector2 = [x2-x1 y2-y1];
        hvector1 = [x1-x2 y1-y2];
        thetaq1 = floor((theta1-0)/1) + 1;
        thetaq2 = floor((theta2-0)/1) + 1;
        Rq1 = floor((R-1)/0.01) + 1;
        Rq2 = floor((R-1)/0.01) + 1;

        % drag fit
        dfz1 = (coefficient_dragq(thetaq1, Rq1) - 1)*fz1;
        dfz2 = (coefficient_dragq(thetaq2, Rq2) - 1)*fz2;

        % sideforce fit
        if norm(hvector1) == 0 % no sideforce
            dfx1 = 0;
            dfy1 = 0;
            dfx2 = 0;
            dfy2 = 0;
        else
            dsideforce1 = coefficient_sideforceq(thetaq1, Rq1)*fz1*hvector1/norm(hvector1);
            dsideforce2 = coefficient_sideforceq(thetaq2, Rq2)*fz2*hvector2/norm(hvector2);
            dfx1 = dsideforce1(1);
            dfy1 = dsideforce1(2);
            dfx2 = dsideforce2(1);
            dfy2 = dsideforce2(2);
        end
    end
end

== matlab function simulink_4_balloons/coupling/Coupling Each two 24/coupling each two ==
  data: x1 input; dfx1 output; y1 input; dfy1 output; dfz1 output; dfx2 output; dfy2 output; dfz2 output; z1 input; fz1 input; x2 input; y2 input; z2 input; fz2 input; rb input; coefficient_dragq input; coefficient_sideforceq input
function [dfx1,dfy1,dfz1,dfx2,dfy2,dfz2] = fcn(x1, y1, z1, fz1, x2, y2, z2, fz2, rb, coefficient_dragq, coefficient_sideforceq)
    % set vector between balloons and z axis
    vector = [x2-x1 y2-y1 z2-z1];
    vectorz = [0 0 1];
    % distance of balloons
    R = norm(vector)/rb/2;
    
    if R >5 || R < 1 % too far
        dfx1 = 0;
        dfy1 = 0;
        dfz1 = 0;
        dfx2 = 0;
        dfy2 = 0;
        dfz2 = 0;
    else % fit curves
        theta2 = acos(dot(vector,vectorz)/(norm(vector)*norm(vectorz)))/pi*180;
        theta1 = 180 - theta2;
        hvector2 = [x2-x1 y2-y1];
        hvector1 = [x1-x2 y1-y2];
        thetaq1 = floor((theta1-0)/1) + 1;
        thetaq2 = floor((theta2-0)/1) + 1;
        Rq1 = floor((R-1)/0.01) + 1;
        Rq2 = floor((R-1)/0.01) + 1;

        % drag fit
        dfz1 = (coefficient_dragq(thetaq1, Rq1) - 1)*fz1;
        dfz2 = (coefficient_dragq(thetaq2, Rq2) - 1)*fz2;

        % sideforce fit
        if norm(hvector1) == 0 % no sideforce
            dfx1 = 0;
            dfy1 = 0;
            dfx2 = 0;
            dfy2 = 0;
        else
            dsideforce1 = coefficient_sideforceq(thetaq1, Rq1)*fz1*hvector1/norm(hvector1);
            dsideforce2 = coefficient_sideforceq(thetaq2, Rq2)*fz2*hvector2/norm(hvector2);
            dfx1 = dsideforce1(1);
            dfy1 = dsideforce1(2);
            dfx2 = dsideforce2(1);
            dfy2 = dsideforce2(2);
        end
    end
end

== matlab function simulink_4_balloons/coupling/Coupling Each two 34/coupling each two ==
  data: x1 input; dfx1 output; y1 input; dfy1 output; dfz1 output; dfx2 output; dfy2 output; dfz2 output; z1 input; fz1 input; x2 input; y2 input; z2 input; fz2 input; rb input; coefficient_dragq input; coefficient_sideforceq input
function [dfx1,dfy1,dfz1,dfx2,dfy2,dfz2] = fcn(x1, y1, z1, fz1, x2, y2, z2, fz2, rb, coefficient_dragq, coefficient_sideforceq)
    % set vector between balloons and z axis
    vector = [x2-x1 y2-y1 z2-z1];
    vectorz = [0 0 1];
    % distance of balloons
    R = norm(vector)/rb/2;
    
    if R >5 || R < 1 % too far
        dfx1 = 0;
        dfy1 = 0;
        dfz1 = 0;
        dfx2 = 0;
        dfy2 = 0;
        dfz2 = 0;
    else % fit curves
        theta2 = acos(dot(vector,vectorz)/(norm(vector)*norm(vectorz)))/pi*180;
        theta1 = 180 - theta2;
        hvector2 = [x2-x1 y2-y1];
        hvector1 = [x1-x2 y1-y2];
        thetaq1 = floor((theta1-0)/1) + 1;
        thetaq2 = floor((theta2-0)/1) + 1;
        Rq1 = floor((R-1)/0.01) + 1;
        Rq2 = floor((R-1)/0.01) + 1;

        % drag fit
        dfz1 = (coefficient_dragq(thetaq1, Rq1) - 1)*fz1;
        dfz2 = (coefficient_dragq(thetaq2, Rq2) - 1)*fz2;

        % sideforce fit
        if norm(hvector1) == 0 % no sideforce
            dfx1 = 0;
            dfy1 = 0;
            dfx2 = 0;
            dfy2 = 0;
        else
            dsideforce1 = coefficient_sideforceq(thetaq1, Rq1)*fz1*hvector1/norm(hvector1);
            dsideforce2 = coefficient_sideforceq(thetaq2, Rq2)*fz2*hvector2/norm(hvector2);
            dfx1 = dsideforce1(1);
            dfy1 = dsideforce1(2);
            dfx2 = dsideforce2(1);
            dfy2 = dsideforce2(2);
        end
    end
end

== matlab function simulink_4_balloons/Subsystem2/Vertical dynamics ==
  data: fx output; sx output; fy output; sy output; x input; xdot input; y input; ydot input; z input; fz output; zdot input; parameters input; sz output
function [fx,sx,fy,sy,fz,sz] = fcn(x,xdot,y,ydot,z,zdot,parameters)

Cd = parameters(1);
rb = parameters(2);
rn = parameters(3);
theta = deg2rad(parameters(4)); 
V0 = parameters(5); 
normalScaling = parameters(6); 

%% Vertical forces

%flow radius
rFlow = rn+z*tan(theta);

%Peak flow velocity
meanFlowVelocity = V0*rn^2/(rFlow)^2;

%Velocity under ball
vFlowActual = flowSpeed(meanFlowVelocity,normalScaling*rFlow,x,y);

%Relative
relativeVelocity = vFlowActual - zdot;

%Force
fz = sign(relativeVelocity)*0.5*Cd*pi*rb^2*1.22*relativeVelocity^2;



%% Horizontal XY forces
% Bernoulli's Principle
if x == 0 && y == 0
    fx = 0;
    fy = 0;
else
    direction = [x y];
    distance = norm(direction);
    one_direction = direction/distance;
    inner_position = (distance - rb)*one_direction;
    outer_position = (distance + rb)*one_direction;
    vInner = flowSpeed(meanFlowVelocity,normalScaling*rFlow,inner_position(1),inner_position(2));
    vOuter = flowSpeed(meanFlowVelocity,normalScaling*rFlow,outer_position(1),outer_position(2));
    fH = 0.5*1.22*(vOuter^2 - vInner^2)*pi*rb^2*one_direction;
    fx = fH(1);
    fy = fH(2);
end
% Drag
if xdot == 0 && ydot == 0
else
    vxy = [xdot ydot];
    dragH = 0.5*Cd*pi*rb^2*1.22*(xdot^2 + ydot^2)*vxy/norm(vxy);
    fx = fx - dragH(1);
    fy = fy - dragH(2);
end

%% Force scalings
sx = flowSpeed(meanFlowVelocity,normalScaling*rFlow,x,0)/flowSpeed(meanFlowVelocity,rFlow,0,0);
sy = flowSpeed(meanFlowVelocity,normalScaling*rFlow,0,y)/flowSpeed(meanFlowVelocity,rFlow,0,0);
sz = flowSpeed(meanFlowVelocity,normalScaling*rFlow,x,y)/flowSpeed(meanFlowVelocity,rFlow,0,0);

== matlab function simulink_4_balloons/Subsystem1/Vertical dynamics ==
  data: fx output; sx output; fy output; sy output; x input; xdot input; y input; ydot input; z input; fz output; zdot input; parameters input; sz output
function [fx,sx,fy,sy,fz,sz] = fcn(x,xdot,y,ydot,z,zdot,parameters)

Cd = parameters(1);
rb = parameters(2);
rn = parameters(3);
theta = deg2rad(parameters(4)); 
V0 = parameters(5); 
normalScaling = parameters(6); 

%% Vertical forces

%flow radius
rFlow = rn+z*tan(theta);

%Peak flow velocity
meanFlowVelocity = V0*rn^2/(rFlow)^2;

%Velocity under ball
vFlowActual = flowSpeed(meanFlowVelocity,normalScaling*rFlow,x,y);

%Relative
relativeVelocity = vFlowActual - zdot;

%Force
fz = sign(relativeVelocity)*0.5*Cd*pi*rb^2*1.22*relativeVelocity^2;



%% Horizontal XY forces
% Bernoulli's Principle
if x == 0 && y == 0
    fx = 0;
    fy = 0;
else
    direction = [x y];
    distance = norm(direction);
    one_direction = direction/distance;
    inner_position = (distance - rb)*one_direction;
    outer_position = (distance + rb)*one_direction;
    vInner = flowSpeed(meanFlowVelocity,normalScaling*rFlow,inner_position(1),inner_position(2));
    vOuter = flowSpeed(meanFlowVelocity,normalScaling*rFlow,outer_position(1),outer_position(2));
    fH = 0.5*1.22*(vOuter^2 - vInner^2)*pi*rb^2*one_direction;
    fx = fH(1);
    fy = fH(2);
end
% Drag
if xdot == 0 && ydot == 0
else
    vxy = [xdot ydot];
    dragH = 0.5*Cd*pi*rb^2*1.22*(xdot^2 + ydot^2)*vxy/norm(vxy);
    fx = fx - dragH(1);
    fy = fy - dragH(2);
end

%% Force scalings
sx = flowSpeed(meanFlowVelocity,normalScaling*rFlow,x,0)/flowSpeed(meanFlowVelocity,rFlow,0,0);
sy = flowSpeed(meanFlowVelocity,normalScaling*rFlow,0,y)/flowSpeed(meanFlowVelocity,rFlow,0,0);
sz = flowSpeed(meanFlowVelocity,normalScaling*rFlow,x,y)/flowSpeed(meanFlowVelocity,rFlow,0,0);

== matlab function simulink_4_balloons/coupling/Coupling Each two 12/coupling each two ==
  data: x1 input; dfx1 output; y1 input; dfy1 output; dfz1 output; dfx2 output; dfy2 output; dfz2 output; z1 input; fz1 input; x2 input; y2 input; z2 input; fz2 input; rb input; coefficient_dragq input; coefficient_sideforceq input
function [dfx1,dfy1,dfz1,dfx2,dfy2,dfz2] = fcn(x1, y1, z1, fz1, x2, y2, z2, fz2, rb, coefficient_dragq, coefficient_sideforceq)
    % set vector between balloons and z axis
    vector = [x2-x1 y2-y1 z2-z1];
    vectorz = [0 0 1];
    % distance of balloons
    R = norm(vector)/rb/2;
    
    if R >5 || R < 1 % too far
        dfx1 = 0;
        dfy1 = 0;
        dfz1 = 0;
        dfx2 = 0;
        dfy2 = 0;
        dfz2 = 0;
    else % fit curves
        theta2 = acos(dot(vector,vectorz)/(norm(vector)*norm(vectorz)))/pi*180;
        theta1 = 180 - theta2;
        hvector2 = [x2-x1 y2-y1];
        hvector1 = [x1-x2 y1-y2];
        thetaq1 = floor((theta1-0)/1) + 1;
        thetaq2 = floor((theta2-0)/1) + 1;
        Rq1 = floor((R-1)/0.01) + 1;
        Rq2 = floor((R-1)/0.01) + 1;

        % drag fit
        dfz1 = (coefficient_dragq(thetaq1, Rq1) - 1)*fz1;
        dfz2 = (coefficient_dragq(thetaq2, Rq2) - 1)*fz2;

        % sideforce fit
        if norm(hvector1) == 0 % no sideforce
            dfx1 = 0;
            dfy1 = 0;
            dfx2 = 0;
            dfy2 = 0;
        else
            dsideforce1 = coefficient_sideforceq(thetaq1, Rq1)*fz1*hvector1/norm(hvector1);
            dsideforce2 = coefficient_sideforceq(thetaq2, Rq2)*fz2*hvector2/norm(hvector2);
            dfx1 = dsideforce1(1);
            dfy1 = dsideforce1(2);
            dfx2 = dsideforce2(1);
            dfy2 = dsideforce2(2);
        end
    end
end

== matlab function simulink_4_balloons/Subsystem3/Vertical dynamics ==
  data: fx output; sx output; fy output; sy output; x input; xdot input; y input; ydot input; z input; fz output; zdot input; parameters input; sz output
function [fx,sx,fy,sy,fz,sz] = fcn(x,xdot,y,ydot,z,zdot,parameters)

Cd = parameters(1);
rb = parameters(2);
rn = parameters(3);
theta = deg2rad(parameters(4)); 
V0 = parameters(5); 
normalScaling = parameters(6); 

%% Vertical forces

%flow radius
rFlow = rn+z*tan(theta);

%Peak flow velocity
meanFlowVelocity = V0*rn^2/(rFlow)^2;

%Velocity under ball
vFlowActual = flowSpeed(meanFlowVelocity,normalScaling*rFlow,x,y);

%Relative
relativeVelocity = vFlowActual - zdot;

%Force
fz = sign(relativeVelocity)*0.5*Cd*pi*rb^2*1.22*relativeVelocity^2;



%% Horizontal XY forces
% Bernoulli's Principle
if x == 0 && y == 0
    fx = 0;
    fy = 0;
else
    direction = [x y];
    distance = norm(direction);
    one_direction = direction/distance;
    inner_position = (distance - rb)*one_direction;
    outer_position = (distance + rb)*one_direction;
    vInner = flowSpeed(meanFlowVelocity,normalScaling*rFlow,inner_position(1),inner_position(2));
    vOuter = flowSpeed(meanFlowVelocity,normalScaling*rFlow,outer_position(1),outer_position(2));
    fH = 0.5*1.22*(vOuter^2 - vInner^2)*pi*rb^2*one_direction;
    fx = fH(1);
    fy = fH(2);
end
% Drag
if xdot == 0 && ydot == 0
else
    vxy = [xdot ydot];
    dragH = 0.5*Cd*pi*rb^2*1.22*(xdot^2 + ydot^2)*vxy/norm(vxy);
    fx = fx - dragH(1);
    fy = fy - dragH(2);
end

%% Force scalings
sx = flowSpeed(meanFlowVelocity,normalScaling*rFlow,x,0)/flowSpeed(meanFlowVelocity,rFlow,0,0);
sy = flowSpeed(meanFlowVelocity,normalScaling*rFlow,0,y)/flowSpeed(meanFlowVelocity,rFlow,0,0);
sz = flowSpeed(meanFlowVelocity,normalScaling*rFlow,x,y)/flowSpeed(meanFlowVelocity,rFlow,0,0);
